simulink model "hop3s"  (R2020b)
settings: Solver=VariableStepAuto  StartTime=0.0  StopTime=150  RelTol=1e-3
libraries: simulink x2
settings Model: Creator=stefanopanzieri  LastModifiedBy=Stefano

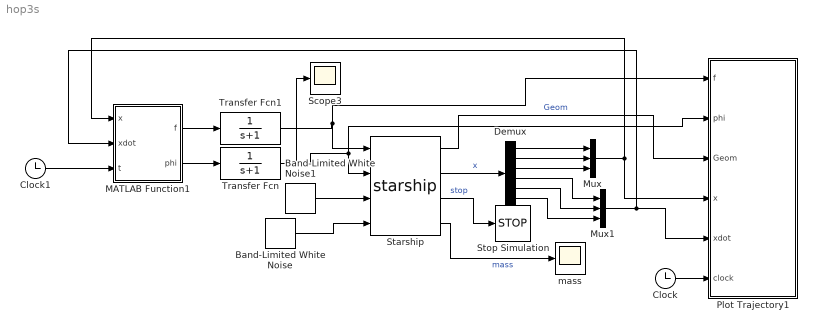
== system hop3s ==
  Band-Limited White Noise : simulink/Sources/Band-Limited White Noise  Cov=[0.00001]  Ts=0.1  seed=[23341]
  Band-Limited White Noise1 : simulink/Sources/Band-Limited White Noise  Cov=[0.000000001]  Ts=0.1  seed=[23341]
  Clock : Clock
  Clock1 : Clock
  Demux : Demux  Outputs=6
  MATLAB Function1 : MATLAB Function  TreatAsAtomicUnit=on
  Mux : Mux  Inputs=3
  Mux1 : Mux  Inputs=3
  Plot Trajectory1 : MATLAB Function  TreatAsAtomicUnit=on  SystemSampleTime=0.1
  Scope3 : Scope
  Starship : M-S-Function  FunctionName=starship  Parameters=0.01
  Stop Simulation : Stop
  Transfer Fcn : TransferFcn  Denominator=[1 1]
  Transfer Fcn1 : TransferFcn  Denominator=[1 1]
  mass : Scope
  wires:
  Clock/1 -> Plot Trajectory1/6(clock)
  Transfer Fcn/1 -> Scope3/1, Starship/2, Plot Trajectory1/2(phi)
  Transfer Fcn1/1 -> Starship/1, Plot Trajectory1/1(f)
  MATLAB Function1/1(f) -> Transfer Fcn1/1
  Clock1/1 -> MATLAB Function1/3(t)
  Band-Limited White Noise1/1 -> Starship/3
  Band-Limited White Noise/1 -> Starship/4
  MATLAB Function1/2(phi) -> Transfer Fcn/1
  Starship/2 -> Demux/1  "x"
  Demux/1 -> Mux/1
  Demux/2 -> Mux/2
  Demux/3 -> Mux/3
  Demux/4 -> Mux1/1
  Demux/5 -> Mux1/2
  Demux/6 -> Mux1/3
  Starship/1 -> Plot Trajectory1/3(Geom)  "Geom"
  Mux/1 -> Plot Trajectory1/4(x), MATLAB Function1/1(x)
  Mux1/1 -> MATLAB Function1/2(xdot), Plot Trajectory1/5(xdot)
  Starship/3 -> Stop Simulation/1  "stop"
  Starship/4 -> mass/1  "mass"

== matlab function hop3s/Plot Trajectory1 ==
  settings: updateMethod=DISCRETE
  data: f input; phi input; Geom input; x input; xdot input; clock input
function PlotRocket(f,phi,Geom,x,xdot,clock)

eml.extrinsic('findobj','get','set','figure','clf',...
              'hold','delete','plot','axis','grid',...
              'hggroup','quiver','drawnow','string');
          
persistent chain;
persistent thrust;
persistent ground;
persistent deleted_fig;

L=Geom(1);
Alt=Geom(2);
Dia=Geom(3);

% posizione del propulsore
pex=x(1)+L*sin(x(3));
pey=x(2)-L*cos(x(3));

% Vettore di propulsione
vex=f*sin(x(3)+phi)/5000;
vey=-f*cos(x(3)+phi)/5000;

          
% Gestisco la figura di output
if isempty(deleted_fig)
    deleted_fig=1;
    % La prima volta cancello la figura
    foundFig=findobj('Tag','trajScope');
    if ~isempty(foundFig)
        cla(foundFig)
        %foundFig=findobj('Tag','stroboScope');
    end      
else
    foundFig=findobj('Tag','trajScope');
end



if isempty(foundFig)
    fig=figure('Color','white');
    clf(fig);
    set(fig,'Name','Trajectory');
    set(fig,'DoubleBuffer','on','Tag','trajScope');
    set(fig,'Renderer','painters');
    hold('on');
    hax=get(fig,'CurrentAxes');
    set(hax,'DrawMode','fast','Box','off');    
    

    chain=hggroup;
    thrust=hggroup; %quiver(hax,pex,pey,vex,vey,'Color','green','LineWidth',2);
    %ground=plot([-30 30],[0 0],'c','LineWidth',3);
    grid('on');
    
else
    
    hax=get(foundFig,'CurrentAxes');

end


if ~isempty(chain)
    delete(chain);
end
    
if ~isempty(thrust)    
    delete(thrust);
end



% draw the center of mass
chain=hggroup;
h1=plot(hax,x(1),x(2),'r*','LineWidth',3);


width = Dia; % whatever
height = (Alt-L)*2/3; % whatever...
xLeft = - width/2;
xRigth = width/2;
yBottom = - L;
yTop = height;
xPoint=0;
yPoint=height*3/2;

Vertex=[xLeft yTop  1
        xPoint yPoint 1
        xRigth yTop  1
        xRigth yBottom 1
        xLeft  yBottom 1
        xLeft yTop  1];
    
Rot=[cos(-x(3))  sin(-x(3)) x(1)
     -sin(-x(3)) cos(-x(3)) x(2)
      0         0        1];
      
Vertex=(Rot*Vertex')';

h2=line(Vertex(:,1),Vertex(:,2));


%h2=rectangle('Position', [xLeft, yBottom, width, height], 'EdgeColor', 'b', 'FaceColor', 'r', 'LineWidth', 4);

set(h1,'Parent',chain);
set(h2,'Parent',chain);



% draw the thrust

thrust=quiver(hax,pex,pey,vex,vey,'Color','green','LineWidth',2);


% draw the ground
if x(2)<100
    if isempty(ground)
        ground=plot([-30 30],[0 0],'c','LineWidth',3);
    end
end



%axis([-2 42 0 102])
xlabel(['vert speed (m/s):' string(xdot(2))])
axis equal
drawnow;

== matlab function hop3s/MATLAB Function1 ==
  data: x input; f output; xdot input; t input; phi output
function [f,phi] = fcn(x,xdot,t)
y=x(1);
z=x(2);
theta=x(3);
ydot=xdot(1);
zdot=xdot(2);
thetadot=xdot(3);


% Proporzionale derivativo che tende a mantenere theta=0;
Kp=4;
Kd=10;
phi=Kp*theta+Kd*xdot(3);

% Reazione dallo stato che mantiene theta=0 e y=0
K=[-0.0057    1.3992   -0.0362    2.4762];
phi=K*[y theta ydot thetadot]';


if t<20
    f=900000;
else
   % valore di riferimento per la velocità
   v_des=-x(2)/30;
   % Controllo proporzionale
   f=200000*(v_des-xdot(2)); 
end


if f<0
    f=0;
end
